simulink model "declarations"  (R2020a)
settings: Solver=VariableStepAuto  StartTime=0.0  StopTime=10.0  RelTol=1e-3
settings Model: Creator=shrad  LastModifiedBy=shrad

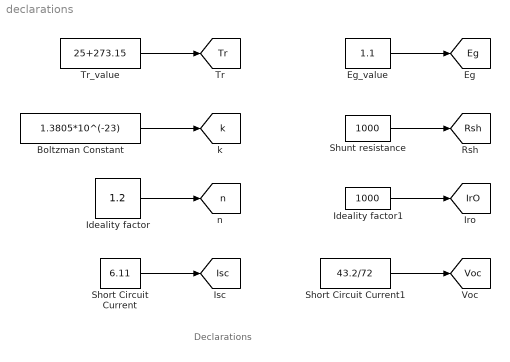
== system declarations ==
  note: Declarations
  Boltzman Constant : Constant  Value=1.3805*10^(-23)
  Eg_value : Constant  Value=1.1
  Ideality factor : Constant  Value=1.2
  Ideality factor1 : Constant  Value=1000
  Short Circuit Current : Constant  Value=6.11
  Short Circuit Current1 : Constant  Value=43.2/72
  Shunt resistance : Constant  Value=1000
  Tr_value : Constant  Value=25+273.15
  tag scope: Eg=global, IrO=global, Isc=global, Rsh=global, Tr=global, Voc=global, k=global, n=global
  wires:
  Shunt resistance/1 -> [Rsh]
  Ideality factor1/1 -> [IrO]
  Eg_value/1 -> [Eg]
  Short Circuit Current1/1 -> [Voc]
  Short Circuit Current/1 -> [Isc]
  Ideality factor/1 -> [n]
  Boltzman Constant/1 -> [k]
  Tr_value/1 -> [Tr]
